simulink library "hostLib"  (R2014b)
settings: Solver=ode45  StartTime=0.0  StopTime=10.0  RelTol=1e-3
settings Model: Creator=scastro  LastModifiedBy=scastro

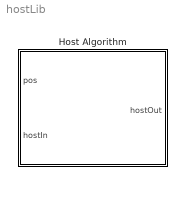
== system hostLib ==
  Host Algorithm : Stateflow chart  TreatAsAtomicUnit=on

== stateflow chart hostLib/Host Algorithm ==
  (default) -> (junction 2) : {hostOut = hostIn;}
  data: pos input; hostIn input; hostOut output
